simulink model "Assignment4"  (R2020b)
settings: Solver=VariableStepAuto  StartTime=0.0  StopTime=10.0  RelTol=1e-3
values from neighbouring files (symbols this model uses):
  A = [0 1; -5 -2]    [Assignment4.m]    (also in Lecture14_LSF.m = [0 1; -1 -2]; Lecture15_DigitalLSF.m = [0 1; -1 -2]; Lecture16_LSFIntegrator.m = [0 1; -1 -2]; Lecture6_3PhaseCurrent.m = 20)
  B = [0; 1]    [Assignment4.m]    (also in Lecture14_LSF.m; Lecture15_DigitalLSF.m; Lecture16_LSFIntegrator.m; dSpaceLab.m = [0; 1/La])
  C = [5 0]    [Assignment4.m]    (also in Lecture14_LSF.m = [10 0]; Lecture15_DigitalLSF.m = [10 0]; Lecture16_LSFIntegrator.m = [10 0]; dSpaceLab.m = [1, 0])
  Cd = C    [Assignment4.m]    (also in Lecture15_DigitalLSF.m)
  K12 = [K(1) K(2)]    [Assignment4.m]    (also in Lecture16_LSFIntegrator.m)
  K_100_12 = [K_100(1) K_100(2)]    [Assignment4.m]
  K_100_i = -K_100(3)    [Assignment4.m]
  K_10_12 = [K_10(1) K_10(2)]    [Assignment4.m]
  K_10_i = -K_10(3)    [Assignment4.m]
  Ki = 1/2    (= 0.5)    [Assignment3.m]    (also in Assignment4.m = -K(3); Lecture13_PolePlacement.m = 0.0125; Lecture16_LSFIntegrator.m = -K(3); Lecture4_DiscretePID.m = 0.8)
  T_100Hz = 1/100    (= 0.01)    [Assignment4.m]
  T_10Hz = 1/10    (= 0.1)    [Assignment4.m]
undefined symbols (not defined in the file or in its folder): Ad_10, Ad_100, Bd_10, Bd_100
settings Model: Creator=sebastian  LastModifiedBy=sebastian

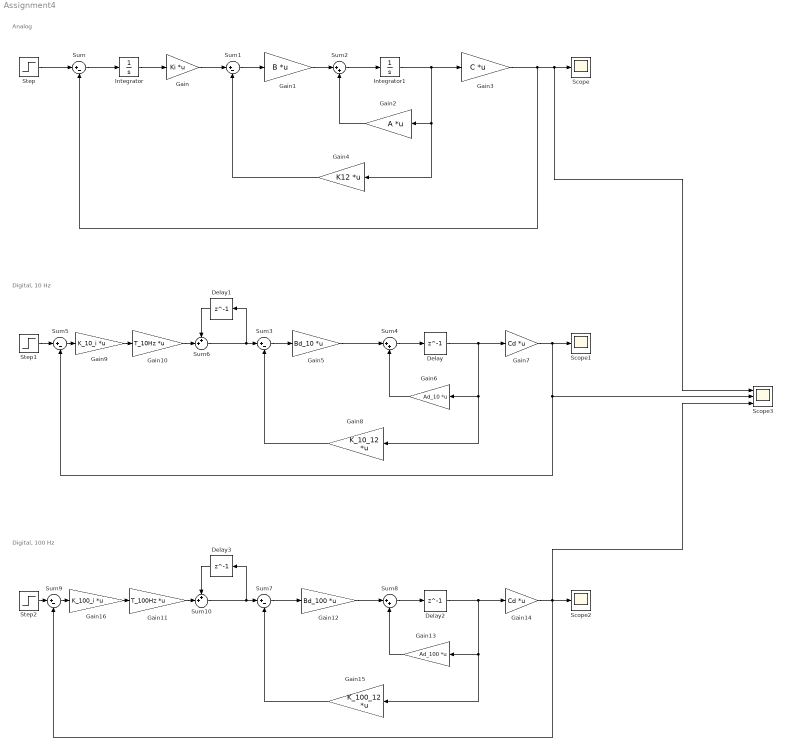
== system Assignment4 ==
  note: Analog
  note: Digital, 10 Hz
  note: Digital, 100 Hz
  Delay : Delay  DelayLength=1  InitialCondition=0  SampleTime=T_10Hz
  Delay1 : Delay  DelayLength=1  SampleTime=T_10Hz
  Delay2 : Delay  DelayLength=1  InitialCondition=0  SampleTime=T_100Hz
  Delay3 : Delay  DelayLength=1  SampleTime=T_100Hz
  Gain : Gain  Gain=Ki  Multiplication=Matrix(K*u)
  Gain1 : Gain  Gain=B  Multiplication=Matrix(K*u)
  Gain10 : Gain  Gain=T_10Hz  Multiplication=Matrix(K*u)
  Gain11 : Gain  Gain=T_100Hz  Multiplication=Matrix(K*u)
  Gain12 : Gain  Gain=Bd_100  Multiplication=Matrix(K*u)
  Gain13 : Gain  Gain=Ad_100  Multiplication=Matrix(K*u)
  Gain14 : Gain  Gain=Cd  Multiplication=Matrix(K*u)
  Gain15 : Gain  Gain=K_100_12  Multiplication=Matrix(K*u)
  Gain16 : Gain  Gain=K_100_i  Multiplication=Matrix(K*u)
  Gain2 : Gain  Gain=A  Multiplication=Matrix(K*u)
  Gain3 : Gain  Gain=C  Multiplication=Matrix(K*u)
  Gain4 : Gain  Gain=K12  Multiplication=Matrix(K*u)
  Gain5 : Gain  Gain=Bd_10  Multiplication=Matrix(K*u)
  Gain6 : Gain  Gain=Ad_10  Multiplication=Matrix(K*u)
  Gain7 : Gain  Gain=Cd  Multiplication=Matrix(K*u)
  Gain8 : Gain  Gain=K_10_12  Multiplication=Matrix(K*u)
  Gain9 : Gain  Gain=K_10_i  Multiplication=Matrix(K*u)
  Integrator : Integrator
  Integrator1 : Integrator
  Scope : Scope
  Scope1 : Scope
  Scope2 : Scope
  Scope3 : Scope  NumInputPorts=3
  Step : Step  SampleTime=0
  Step1 : Step  SampleTime=0
  Step2 : Step  SampleTime=0
  Sum{,1,3,5,7,9} (6 alike) : Sum  Inputs=|+-
  Sum10 : Sum  Inputs=++|
  Sum2 : Sum  Inputs=|++
  Sum4 : Sum  Inputs=|++
  Sum6 : Sum  Inputs=++|
  Sum8 : Sum  Inputs=|++
  wires:
  Gain3/1 -> Sum/2, Scope3/1, Scope/1
  Integrator1/1 -> Gain4/1, Gain2/1, Gain3/1
  Step/1 -> Sum/1
  Gain4/1 -> Sum1/2
  Integrator/1 -> Gain/1
  Gain2/1 -> Sum2/2
  Sum1/1 -> Gain1/1
  Sum/1 -> Integrator/1
  Sum2/1 -> Integrator1/1
  Gain/1 -> Sum1/1
  Gain1/1 -> Sum2/1
  Gain5/1 -> Sum4/1
  Sum4/1 -> Delay/1
  Sum3/1 -> Gain5/1
  Gain8/1 -> Sum3/2
  Delay/1 -> Gain8/1, Gain6/1, Gain7/1
  Gain6/1 -> Sum4/2
  Gain7/1 -> Scope3/2, Sum5/2, Scope1/1
  Step1/1 -> Sum5/1
  Gain9/1 -> Gain10/1
  Sum5/1 -> Gain9/1
  Gain10/1 -> Sum6/2
  Delay1/1 -> Sum6/1
  Sum6/1 -> Delay1/1, Sum3/1
  Gain15/1 -> Sum7/2
  Gain14/1 -> Scope3/3, Sum9/2, Scope2/1
  Delay2/1 -> Gain15/1, Gain13/1, Gain14/1
  Gain13/1 -> Sum8/2
  Gain16/1 -> Gain11/1
  Step2/1 -> Sum9/1
  Sum8/1 -> Delay2/1
  Gain11/1 -> Sum10/2
  Sum7/1 -> Gain12/1
  Gain12/1 -> Sum8/1
  Sum9/1 -> Gain16/1
  Sum10/1 -> Delay3/1, Sum7/1
  Delay3/1 -> Sum10/1
